simulink model "exam5"  (R2016a)
settings: Solver=VariableStepAuto  StartTime=0.0  StopTime=10.0  RelTol=1e-3
undefined symbols (not defined in the file or in its folder): Kp, N, Td, Ti
settings Model: Creator=linghao  LastModifiedBy=linghao
settings DataIOCC: SaveFormat=Array
settings GRTTargetCC: GeneratePreprocessorConditionals=Use local settings

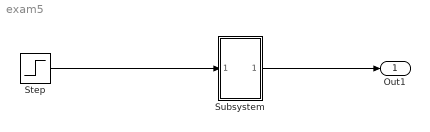
== system exam5 ==
  Step : Step  SampleTime=0
  Subsystem : Subsystem
      mask Display: disp('PID')
  Out1 : Outport
  wires:
  Step/1 -> Subsystem/1(In1)
  Subsystem/1(Out1) -> Out1/1

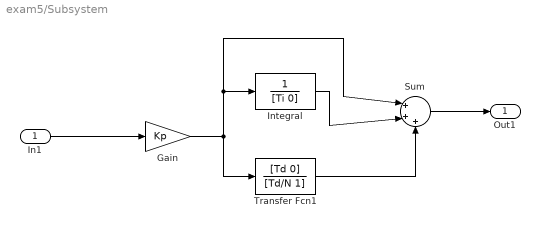
== system exam5/Subsystem ==
  In1 : Inport
  Gain : Gain  Gain=Kp
  "Integral " : TransferFcn  Denominator=[Ti 0]
  Sum : Sum  Inputs=|+++
  Transfer Fcn1 : TransferFcn  Numerator=[Td 0]  Denominator=[Td/N 1]
  Out1 : Outport
  wires:
  Gain/1 -> Transfer Fcn1/1, "Integral "/1, Sum/1
  "Integral "/1 -> Sum/2
  Transfer Fcn1/1 -> Sum/3
  In1/1 -> Gain/1
  Sum/1 -> Out1/1
